simulink model "OneDOF_original"  (Simulink 7.2)
settings: Solver=ode3  StartTime=0.0  StopTime=10.0  FixedStep=10^-3  RelTol=1e-3
values from neighbouring files (symbols this model uses):
  c = zeta*2*m*2*pi*f_vector(i)    [PID_performance_evaluation.m]    (also in PID_surface.m; ResponseSpectrum.m = zeta * 2 * m * 2*pi*f_vector_accel(i); transFunc_2DoF.m)
  k = k+1    (= 2)    [Integra.m]    (also in PID_performance_evaluation.m = m*(2*pi*f_vector(i))^2; PID_surface.m = m*(2*pi*f_vector(i))^2; ResponseSpectrum.m = m * (2*pi*f_vector_accel(i))^2; transFunc_2DoF.m = m*(2*pi*f_vector(i))^2)
  m = (xc1(end,i-1)-xc1(k,i-1))/(Sttime-In(k,1))    [Integra.m]    (also in PID_performance_evaluation.m = 1; PID_surface.m = 1; ResponseSpectrum.m = 1; experimental_setup_possible_freqs.m = 1790)
settings Model: Creator=FVOliveira  LastModifiedBy=FVOliveira
settings DataIOCC: LimitDataPoints=off  SaveFormat=Structure  SaveOutput=off  SignalLogging=off  SaveTime=off
settings DebuggingCC: SolverPrmCheckMsg=none

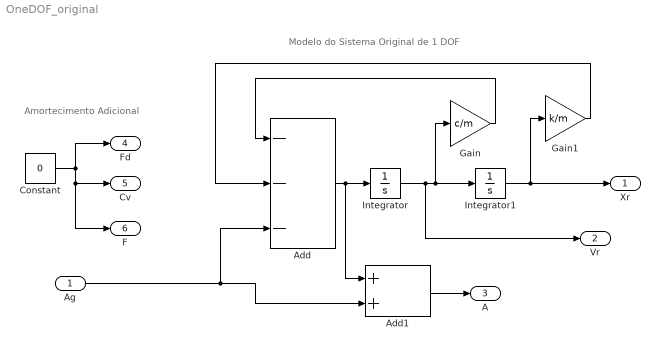
== system OneDOF_original ==
  note: Modelo do Sistema Original de 1 DOF
  note: Amortecimento Adicional
  Ag : Inport  OutDataType=sfix(16)  OutScaling=2^0
  Add : Sum  Inputs=---  OutDataType=sfix(16)  OutScaling=2^-10
  Add1 : Sum  OutDataType=sfix(16)  OutScaling=2^-10
  Constant : Constant  Value=0  OutDataType=sfix(16)  OutScaling=2^0
  Gain : Gain  Gain=c/m  ParameterDataType=sfix(16)  ParameterScaling=2^0  OutDataType=sfix(16)  OutScaling=2^0
  Gain1 : Gain  Gain=k/m  ParameterDataType=sfix(16)  ParameterScaling=2^0  OutDataType=sfix(16)  OutScaling=2^0
  Integrator : Integrator
  Integrator1 : Integrator
  Xr : Outport  OutDataType=sfix(16)  OutScaling=2^0
  Vr : Outport  Port=2  OutDataType=sfix(16)  OutScaling=2^0
  A : Outport  Port=3  OutDataType=sfix(16)  OutScaling=2^0
  Fd : Outport  Port=4  OutDataType=sfix(16)  OutScaling=2^0
  Cv : Outport  Port=5  OutDataType=sfix(16)  OutScaling=2^0
  F : Outport  Port=6  OutDataType=sfix(16)  OutScaling=2^0
  wires:
  Add/1 -> Integrator/1, Add1/1
  Integrator/1 -> Integrator1/1, Gain/1, Vr/1
  Integrator1/1 -> Gain1/1, Xr/1
  Gain1/1 -> Add/2
  Gain/1 -> Add/1
  Add1/1 -> A/1
  Ag/1 -> Add1/2, Add/3
  Constant/1 -> Fd/1, Cv/1, F/1
